simulink model "ControllerSimulation"  (R2022a)
settings: Solver=VariableStepAuto  StartTime=0.0  StopTime=10.0  RelTol=1e-3
undefined symbols (not defined in the file): Kp, Tc, Ti
settings Model: Creator=ykamatan  LastModifiedBy=ykamatan
settings SolverCC: AlgebraicLoopSolver=TrustRegion
settings DebuggingCC: UnconnectedInputMsg=warning  UnconnectedOutputMsg=warning  UnconnectedLineMsg=warning  SFMachineParentedDataDiag=warning
settings RTWCC: DLArmComputeVersion=19.05

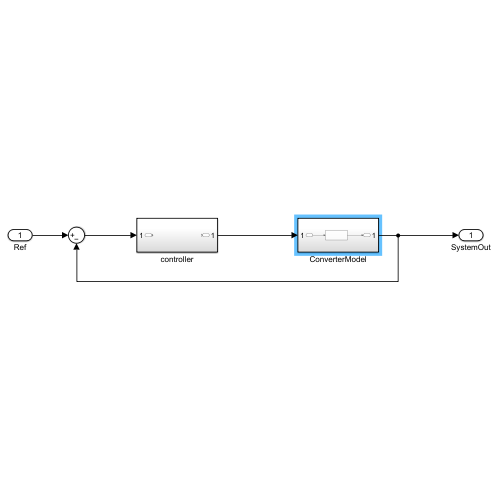
[thumbnail: Simulink's stored preview of the top-level diagram]
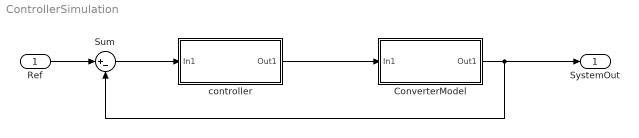
== system ControllerSimulation ==
  Ref : Inport
  ConverterModel : Subsystem
  Sum : Sum  Inputs=|+-
  controller : Subsystem
  SystemOut : Outport
  wires:
  Sum/1 -> controller/1(In1)
  ConverterModel/1(Out1) -> Sum/2, SystemOut/1
  controller/1(Out1) -> ConverterModel/1(In1)
  Ref/1 -> Sum/1

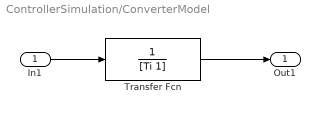
== system ControllerSimulation/ConverterModel ==
  In1 : Inport
  Transfer Fcn : TransferFcn  Denominator=[Ti 1]
  Out1 : Outport
  wires:
  In1/1 -> Transfer Fcn/1
  Transfer Fcn/1 -> Out1/1

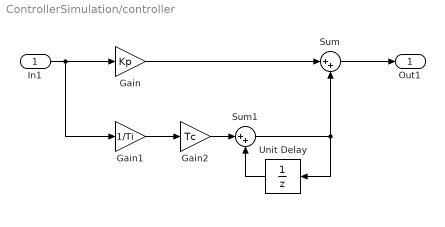
== system ControllerSimulation/controller ==
  In1 : Inport
  Gain : Gain  Gain=Kp
  Gain1 : Gain  Gain=1/Ti
  Gain2 : Gain  Gain=Tc
  Sum : Sum  Inputs=|++
  Sum1 : Sum  Inputs=|++
  Unit Delay : UnitDelay  SampleTime=Tc  HasFrameUpgradeWarning=on
  Out1 : Outport
  wires:
  In1/1 -> Gain1/1, Gain/1
  Gain/1 -> Sum/1
  Sum/1 -> Out1/1
  Gain1/1 -> Gain2/1
  Gain2/1 -> Sum1/1
  Unit Delay/1 -> Sum1/2
  Sum1/1 -> Unit Delay/1, Sum/2
